simulink library "Room_Node"  (R2013b)
settings: Solver=ode45  StartTime=0.0  StopTime=10.0  RelTol=1e-3
undefined symbols (not defined in the file): density, heat_capacity
libraries: simulink x2, simulink_extras x1
settings Model: Creator=lena.frank  LastModifiedBy=drhf

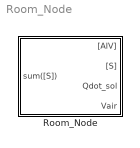
== system Room_Node ==
  Room_Node : Subsystem  mask(NODE){zoneairvolume=5*5*2.5, zoneheight=2.5, zonestartTEMP=20, zonestartWATER=55, timeconst=100, heatperfect=natural, lookuptime=[0 24]*3600, lookupvalue=[20 20], AirPressure=101300}
      mask prompts: zoneairvolume "SIZE: netto air volume >0, m^3"; zoneheight "SIZE: height of zone (floor - ceiling) >0, m"; zonestartTEMP "START TEMPERATURE: convective and radiative node, °C"; zonestartWATER "START AIR HUMIDITY: relative air humidity [0,100], %"; timeconst "timeconstant of radiative and convective node in s"; heatperfect "air temperature"; lookuptime "time vector for ideal profile [s]"; lookupvalue "values for ideal profile [degree centigrade]"; AirPressure "Air pressure for material properties in Pa"
      mask help:
      | This block delivers the energy consumption, temperature and air quality of a zone.
      | It is assumed that this node represents the center of a zone all connected sink and source blocks communicate with. Sink and source blocks are walls, windows, persons, heater etc..
      | Properties of air are calculated once at initialization (with node start temperature, humidity and air pressure).
      | [S] : input vector from sink blocks and source blocks
      | [AIV] : output vector with node temperature and air quality data.
      mask init:
      | CO2norm = 400*1e-6;
      | zoneairvolume = max(0.01, zoneairvolume);
      | zoneheight = max(0.01, zoneheight);
      | zonestartWATER = min(100, max(0, zonestartWATER));
      | zonestartWATER = rel_hum2x(zonestartTEMP, 10^5, zonestartWATER)*1.18*zoneairvolume; % kg H2O in zone volume (at 20°C)
      | zonestartCO2 = CO2norm*1.529*zoneairvolume; % kg CO2 in zone volume
      | zonestartAIR = 10^5*zoneairvolume/(287*(zonestartTEMP+273)); % kg AIR in zone volume
      mask Help: web(fullfile(path_carnot('help'),'Room_Node.html'),'-helpbrowser')
      mask TypeOptions heatperfect: natural | ideal profile (for heating demand)

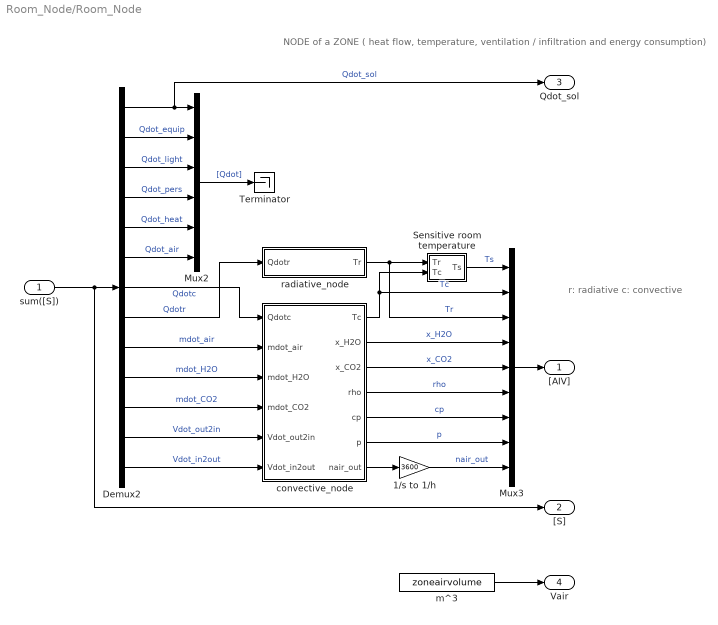
== system Room_Node/Room_Node ==
  note: NODE of a ZONE ( heat flow, temperature, ventilation / infiltration and energy consumption)
  note: r: radiative
      | c: convective
  sum([S]) : Inport
  1/s to 1/h : Gain  Gain=3600  SaturateOnIntegerOverflow=on  OutDataTypeStr=Inherit: Same as input  ParamDataTypeStr=Inherit: Same as input
  Demux2 : Demux  Outputs=13
  Mux2 : Mux  Inputs=6
  Mux3 : Mux  Inputs=9
  Sensitive room temperature : Subsystem  mask(SENSITIVE TEMPERATURE){share_c=47}
      mask prompts: share_c "SHARE of convective sensitivity, [0,100%]:"
      mask help:
      | This block merges the convective and radiative zone node temperature to the SENSITIVE ZONE TEMPERATURE (weighted arithmetic average of both components).
      |
      | [T] = [Tc; Tr]:  temperature vector of node, °C
      | Ts:              sensitive zone temperature, °C
      mask init:
      | blockname = gcb;
      | 
      | if (length(share_c)~=1) error(['PARAMETERS block "' blockname ': "SHARE of ..." must have only 1 entry !']); end;
      | if (share_c<0) | (share_c>100) error(['PARAMETERS block "' blockname '" : "SHARE of ..." must be within [0, 100%] !']); end;
      | share_c = share_c/100;
  Terminator : Terminator
  convective_node : Subsystem
  m^3 : Constant  Value=zoneairvolume
  radiative_node : Subsystem
  "[AIV]" : Outport
  "[S]" : Outport  Port=2
  Qdot_sol : Outport  Port=3
  Vair : Outport  Port=4
  wires:
  Sensitive room temperature/1(Ts) -> Mux3/1  "Ts"
  Mux3/1 -> "[AIV]"/1
  Demux2/13 -> convective_node/6(Vdot_in2out)  "Vdot_in2out"
  Demux2/12 -> convective_node/5(Vdot_out2in)  "Vdot_out2in"
  Demux2/11 -> convective_node/4(mdot_CO2)  "mdot_CO2"
  Demux2/10 -> convective_node/3(mdot_H2O)  "mdot_H2O"
  Demux2/9 -> convective_node/2(mdot_air)  "mdot_air"
  radiative_node/1(Tr) -> Mux3/3, Sensitive room temperature/1(Tr)  "Tr"
  convective_node/1(Tc) -> Mux3/2, Sensitive room temperature/2(Tc)  "Tc"
  convective_node/7(nair_out) -> 1/s to 1/h/1
  convective_node/4(rho) -> Mux3/6  "rho"
  convective_node/5(cp) -> Mux3/7  "cp"
  convective_node/6(p) -> Mux3/8  "p"
  convective_node/3(x_CO2) -> Mux3/5  "x_CO2"
  convective_node/2(x_H2O) -> Mux3/4  "x_H2O"
  1/s to 1/h/1 -> Mux3/9  "nair_out"
  Demux2/1 -> Qdot_sol/1, Mux2/1  "Qdot_sol"
  Demux2/2 -> Mux2/2  "Qdot_equip"
  Demux2/3 -> Mux2/3  "Qdot_light"
  Demux2/4 -> Mux2/4  "Qdot_pers"
  Demux2/5 -> Mux2/5  "Qdot_heat"
  Demux2/6 -> Mux2/6  "Qdot_air"
  Demux2/7 -> convective_node/1(Qdotc)  "Qdotc"
  Demux2/8 -> radiative_node/1(Qdotr)  "Qdotr"
  sum([S])/1 -> Demux2/1, "[S]"/1
  Mux2/1 -> Terminator/1  "[Qdot]"
  m^3/1 -> Vair/1

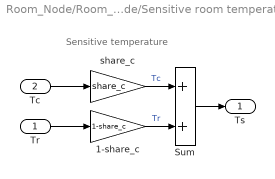
== system Room_Node/Room_Node/Sensitive room temperature ==
  note: Sensitive temperature
  Tr : Inport
  Tc : Inport  Port=2
  1-share_c : Gain  Gain=1-share_c  SaturateOnIntegerOverflow=on  OutDataTypeStr=Inherit: Same as input  ParamDataTypeStr=Inherit: Same as input
  Sum : Sum  SaturateOnIntegerOverflow=on  InputSameDT=on  OutDataTypeStr=Inherit: Same as first input
  share_c : Gain  Gain=share_c  SaturateOnIntegerOverflow=on  OutDataTypeStr=Inherit: Same as input  ParamDataTypeStr=Inherit: Same as input
  Ts : Outport
  wires:
  Tr/1 -> 1-share_c/1
  Tc/1 -> share_c/1
  share_c/1 -> Sum/1  "Tc"
  1-share_c/1 -> Sum/2  "Tr"
  Sum/1 -> Ts/1

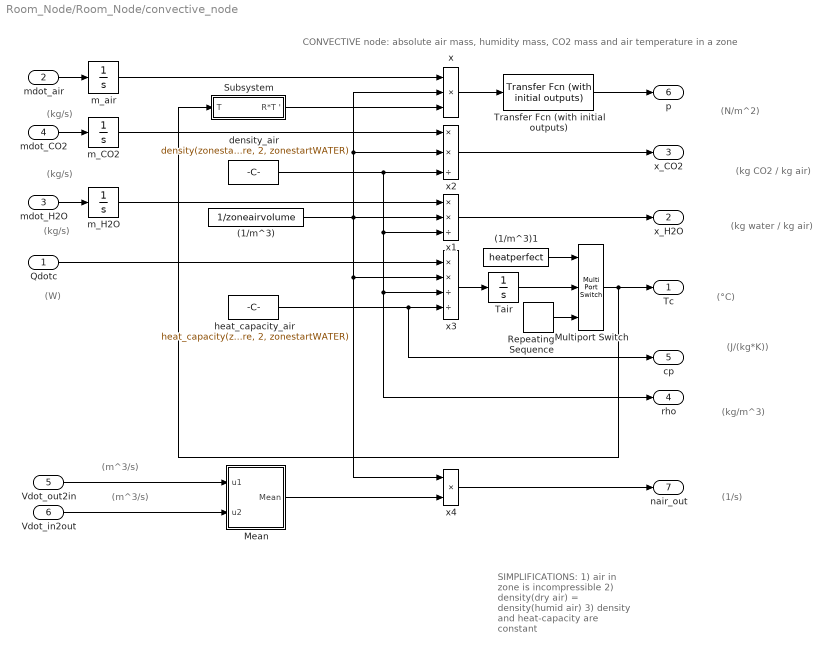
== system Room_Node/Room_Node/convective_node ==
  note: (m^3/s)
  note: (kg/s)
  note: (W)
  note: (°C)
  note: (kg water / kg air)
  note: (kg/s)
  note: (kg/s)
  note: (m^3/s)
  note: (1/s)
  note: CONVECTIVE node: absolute air mass, humidity mass, CO2 mass and air temperature in a zone
  note: (kg/m^3)
  note: SIMPLIFICATIONS:
      | 1) air in zone is incompressible
      | 2) density(dry air) = density(humid air)
      | 3) density and heat-capacity are constant
  note: (J/(kg*K))
  note: (kg CO2 / kg air)
  note: (N/m^2)
  Qdotc : Inport
  mdot_air : Inport  Port=2
  mdot_H2O : Inport  Port=3
  mdot_CO2 : Inport  Port=4
  Vdot_out2in : Inport  Port=5
  Vdot_in2out : Inport  Port=6
  (1/m^3) : Constant  Value=1/zoneairvolume
  (1/m^3)1 : Constant  Value=heatperfect
  Mean : Subsystem
  Multiport Switch : MultiPortSwitch  Inputs=2  SaturateOnIntegerOverflow=on  InputSameDT=on
  Repeating Sequence : simulink/Sources/Repeating Sequence  rep_seq_t=lookuptime  rep_seq_y=lookupvalue
  Subsystem : Subsystem
  Tair : Integrator  InitialCondition=zonestartTEMP
  Transfer Fcn (with initial outputs) : simulink_extras/Additional Linear/Transfer Fcn (with initial outputs)  N=[1]  D=[timeconst 1]  Y0=1e5  U0=0
  density_air : Constant  Value=density(zonestartTEMP, AirPressure, 2, zonestartWATER)
  heat_capacity_air : Constant  Value=heat_capacity(zonestartTEMP, AirPressure, 2, zonestartWATER)
  m_CO2 : Integrator  InitialCondition=zonestartCO2  LimitOutput=on  LowerSaturationLimit=0
  m_H2O : Integrator  InitialCondition=zonestartWATER  LimitOutput=on  LowerSaturationLimit=0
  m_air : Integrator  InitialCondition=zonestartAIR  LimitOutput=on  LowerSaturationLimit=0
  x : Product  Inputs=***  SaturateOnIntegerOverflow=on  InputSameDT=on  OutDataTypeStr=Inherit: Same as first input
  x1 : Product  Inputs=**/  SaturateOnIntegerOverflow=on  InputSameDT=on  OutDataTypeStr=Inherit: Same as first input
  x2 : Product  Inputs=**/  SaturateOnIntegerOverflow=on  InputSameDT=on  OutDataTypeStr=Inherit: Same as first input
  x3 : Product  Inputs=**//  SaturateOnIntegerOverflow=on  InputSameDT=on  OutDataTypeStr=Inherit: Same as first input
  x4 : Product  Inputs=**  SaturateOnIntegerOverflow=on  InputSameDT=on  OutDataTypeStr=Inherit: Same as first input
  Tc : Outport
  x_H2O : Outport  Port=2
  x_CO2 : Outport  Port=3
  rho : Outport  Port=4
  cp : Outport  Port=5
  p : Outport  Port=6
  nair_out : Outport  Port=7
  wires:
  Transfer Fcn (with initial outputs)/1 -> p/1
  density_air/1 -> rho/1, x3/3, x1/3, x2/3
  Qdotc/1 -> x3/1
  Mean/1(Mean) -> x4/2
  Vdot_out2in/1 -> Mean/1(u1)
  Vdot_in2out/1 -> Mean/2(u2)
  x4/1 -> nair_out/1
  x/1 -> Transfer Fcn (with initial outputs)/1
  m_H2O/1 -> x1/1
  mdot_CO2/1 -> m_CO2/1
  mdot_H2O/1 -> m_H2O/1
  x1/1 -> x_H2O/1
  Subsystem/1(R*T ') -> x/3
  mdot_air/1 -> m_air/1
  m_air/1 -> x/1
  heat_capacity_air/1 -> x3/4, cp/1
  m_CO2/1 -> x2/1
  (1/m^3)/1 -> x2/2, x/2, x1/2, x3/2, x4/1
  x3/1 -> Tair/1
  Tair/1 -> Multiport Switch/2
  x2/1 -> x_CO2/1
  Multiport Switch/1 -> Subsystem/1(T), Tc/1
  (1/m^3)1/1 -> Multiport Switch/1
  Repeating Sequence/1 -> Multiport Switch/3

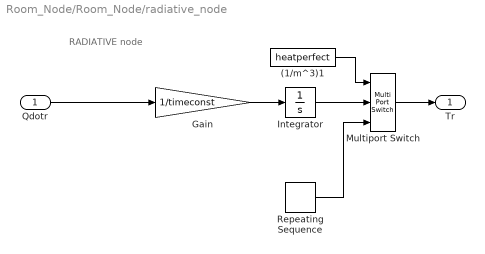
== system Room_Node/Room_Node/radiative_node ==
  note: RADIATIVE node
  Qdotr : Inport
  (1/m^3)1 : Constant  Value=heatperfect
  Gain : Gain  Gain=1/timeconst
  Integrator : Integrator  InitialCondition=zonestartTEMP
  Multiport Switch : MultiPortSwitch  Inputs=2  SaturateOnIntegerOverflow=on  InputSameDT=on
  Repeating Sequence : simulink/Sources/Repeating Sequence  rep_seq_t=lookuptime  rep_seq_y=lookupvalue
  Tr : Outport
  wires:
  Multiport Switch/1 -> Tr/1
  Integrator/1 -> Multiport Switch/2
  (1/m^3)1/1 -> Multiport Switch/1
  Qdotr/1 -> Gain/1
  Gain/1 -> Integrator/1
  Repeating Sequence/1 -> Multiport Switch/3

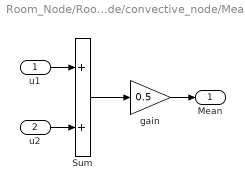
== system Room_Node/Room_Node/convective_node/Mean ==
  u1 : Inport
  u2 : Inport  Port=2
  Sum : Sum  SaturateOnIntegerOverflow=on  InputSameDT=on  OutDataTypeStr=Inherit: Same as first input
  gain : Gain  Gain=0.5  SaturateOnIntegerOverflow=on  OutDataTypeStr=Inherit: Same as input  ParamDataTypeStr=Inherit: Same as input
  Mean : Outport
  wires:
  u2/1 -> Sum/2
  gain/1 -> Mean/1
  u1/1 -> Sum/1
  Sum/1 -> gain/1

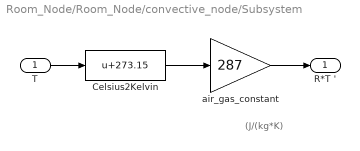
== system Room_Node/Room_Node/convective_node/Subsystem ==
  note: (J/(kg*K)
  T : Inport
  Celsius2Kelvin : Bias  Bias=273.15
  air_gas_constant : Gain  Gain=287  SaturateOnIntegerOverflow=on  OutDataTypeStr=Inherit: Same as input  ParamDataTypeStr=Inherit: Same as input
  R*T ' : Outport
  wires:
  Celsius2Kelvin/1 -> air_gas_constant/1
  T/1 -> Celsius2Kelvin/1
  air_gas_constant/1 -> R*T '/1
